simulink model "untitled"  (R2019b)
settings: Solver=FixedStepAuto  StartTime=0.0  StopTime=10.0  FixedStep=0.05  RelTol=1e-3
settings Model: Creator=51948  LastModifiedBy=51948

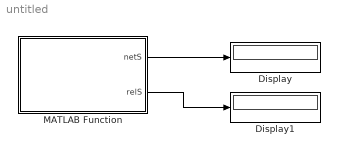
== system untitled ==
  Display : Display
  Display1 : Display
  MATLAB Function : MATLAB Function  TreatAsAtomicUnit=on
  wires:
  MATLAB Function/1(netS) -> Display/1
  MATLAB Function/2(relS) -> Display1/1

== matlab function untitled/MATLAB Function ==
  settings: sampleTime=0.05
  data: netS output size=[2,1]; relS output
function [netS, relS] = predictKA()
%     % 加载训练好的模型
    persistent fnB fnT;
    if isempty(fnB) || isempty(fnT)
        data = load('trainedKAmodel.mat');
        fnB = data.fnB;
        fnT = data.fnT;
    end
    
    
%     m = 6;
%     x = rand(1,m);
    
    % 输入数据归一化（根据训练时的数据范围调整）
    xmin = 0; xmax = 1;
    ymin = 0; ymax = 0.5;
%     
    % 创建一个 3x3 的矩阵
%     dd = zeros(1, 6);  % 初始化为零矩阵
    

    dd = [0.148,0.981,0.425,0.508,0.576,0.353];
    
    
    
    % 使用模型进行预测
    netS = Copy_of_modelKA_basisC( dd, xmin, xmax, ymin, ymax, fnB, fnT );  % 如果使用的是分段线性模型，则改用modelKA_linear
      
    sides = [ sqrt( (dd(:,3)-dd(:,1)).^2 + (dd(:,4)-dd(:,2)).^2 )  sqrt( (dd(:,5)-dd(:,3)).^2 + (dd(:,6)-dd(:,4)).^2 )  sqrt( (dd(:,1)-dd(:,5)).^2 + (dd(:,2)-dd(:,6)).^2 ) ];
    hper = ( sides(:,1) + sides(:,2) + sides(:,3) )/2;
    relS = sqrt( hper .* ( hper - sides(:,1) ) .* ( hper - sides(:,2) ) .* ( hper - sides(:,3) ) );
    
end
